simulink model "Driver"  (R2023b)
settings: Solver=FixedStepAuto  StartTime=0.0  StopTime=10.0  FixedStep=dt  RelTol=1e-3
undefined symbols (not defined in the file): lookAheadDistance, lowpassT, steerLockDeg, torqueLimit, trackReference
libraries: slpidlib x3, simulink_extras x2, eeGeneralControl x1
settings Model: Creator=lukec  LastModifiedBy=lukec

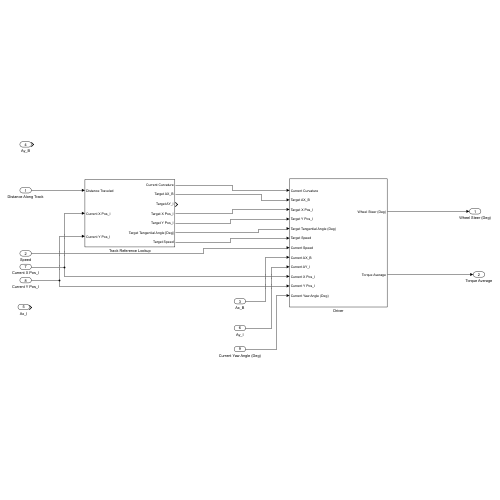
[thumbnail: Simulink's stored preview of the top-level diagram]
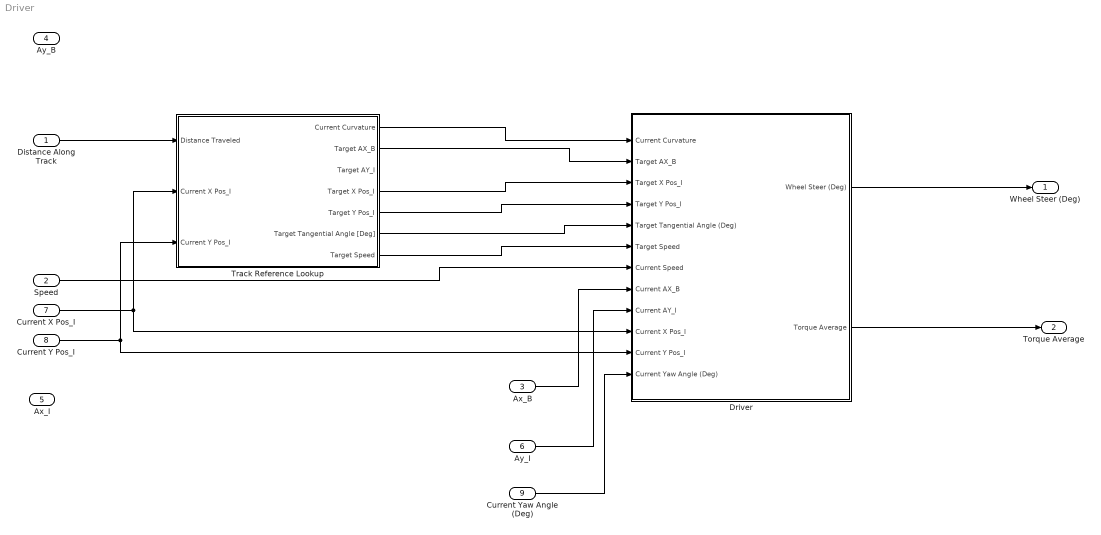
== system Driver ==
  Distance Along Track : Inport
  Speed : Inport  Port=2
  Ax_B : Inport  Port=3
  Ay_B : Inport  Port=4
  Ax_I : Inport  Port=5
  Ay_I : Inport  Port=6
  Current X Pos_I : Inport  Port=7
  Current Y Pos_I : Inport  Port=8
  Current Yaw Angle (Deg) : Inport  Port=9
  Driver : Subsystem
  Track Reference Lookup : Subsystem
  Wheel Steer (Deg) : Outport
  Torque Average : Outport  Port=2
  wires:
  Driver/1(Wheel Steer (Deg)) -> Wheel Steer (Deg)/1
  Track Reference Lookup/1(Current Curvature) -> Driver/1(Current Curvature)
  Track Reference Lookup/2(Target AX_B) -> Driver/2(Target AX_B)
  Track Reference Lookup/4(Target X Pos_I) -> Driver/3(Target X Pos_I)
  Track Reference Lookup/5(Target Y Pos_I) -> Driver/4(Target Y Pos_I)
  Distance Along Track/1 -> Track Reference Lookup/1(Distance Traveled)
  Ax_B/1 -> Driver/8(Current AX_B)
  Ay_I/1 -> Driver/9(Current AY_I)
  Current X Pos_I/1 -> Track Reference Lookup/2(Current X Pos_I), Driver/10(Current X Pos_I)
  Current Y Pos_I/1 -> Track Reference Lookup/3(Current Y Pos_I), Driver/11(Current Y Pos_I)
  Current Yaw Angle (Deg)/1 -> Driver/12(Current Yaw Angle (Deg))
  Track Reference Lookup/6(Target Tangential Angle [Deg]) -> Driver/5(Target Tangential Angle (Deg))
  Speed/1 -> Driver/7(Current Speed)
  Track Reference Lookup/7(Target Speed) -> Driver/6(Target Speed)
  Driver/2(Torque Average) -> Torque Average/1

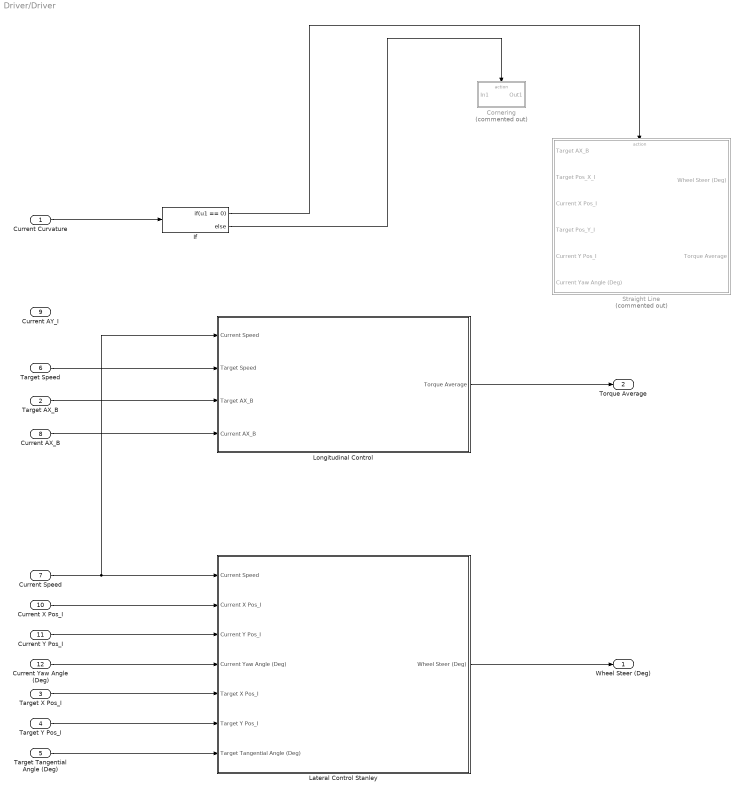
== system Driver/Driver ==
  Current Curvature : Inport
  Target AX_B : Inport  Port=2
  Target X Pos_I : Inport  Port=3
  Target Y Pos_I : Inport  Port=4
  Target Tangential Angle (Deg) : Inport  Port=5
  Target Speed : Inport  Port=6
  Current Speed : Inport  Port=7
  Current AX_B : Inport  Port=8
  Current AY_I : Inport  Port=9
  Current X Pos_I : Inport  Port=10
  Current Y Pos_I : Inport  Port=11
  Current Yaw Angle (Deg) : Inport  Port=12
  Cornering : Subsystem  Commented=on  TreatAsAtomicUnit=on
  If : If  IfExpression=u1 == 0
  Lateral Control Stanley : Subsystem
  Longitudinal Control : Subsystem
  Straight Line : Subsystem  Commented=on  TreatAsAtomicUnit=on
  Wheel Steer (Deg) : Outport
  Torque Average : Outport  Port=2
  wires:
  Current Curvature/1 -> If/1
  If/1 -> Straight Line/Action
  If/2 -> Cornering/Action
  Target X Pos_I/1 -> Lateral Control Stanley/5(Target X Pos_I)
  Target Y Pos_I/1 -> Lateral Control Stanley/6(Target Y Pos_I)
  Current X Pos_I/1 -> Lateral Control Stanley/2(Current X Pos_I)
  Current Y Pos_I/1 -> Lateral Control Stanley/3(Current Y Pos_I)
  Current Yaw Angle (Deg)/1 -> Lateral Control Stanley/4(Current Yaw Angle (Deg))
  Target Tangential Angle (Deg)/1 -> Lateral Control Stanley/7(Target Tangential Angle (Deg))
  Current Speed/1 -> Longitudinal Control/1(Current Speed), Lateral Control Stanley/1(Current Speed)
  Lateral Control Stanley/1(Wheel Steer (Deg)) -> Wheel Steer (Deg)/1
  Longitudinal Control/1(Torque Average) -> Torque Average/1
  Target Speed/1 -> Longitudinal Control/2(Target Speed)
  Current AX_B/1 -> Longitudinal Control/4(Current AX_B)
  Target AX_B/1 -> Longitudinal Control/3(Target AX_B)

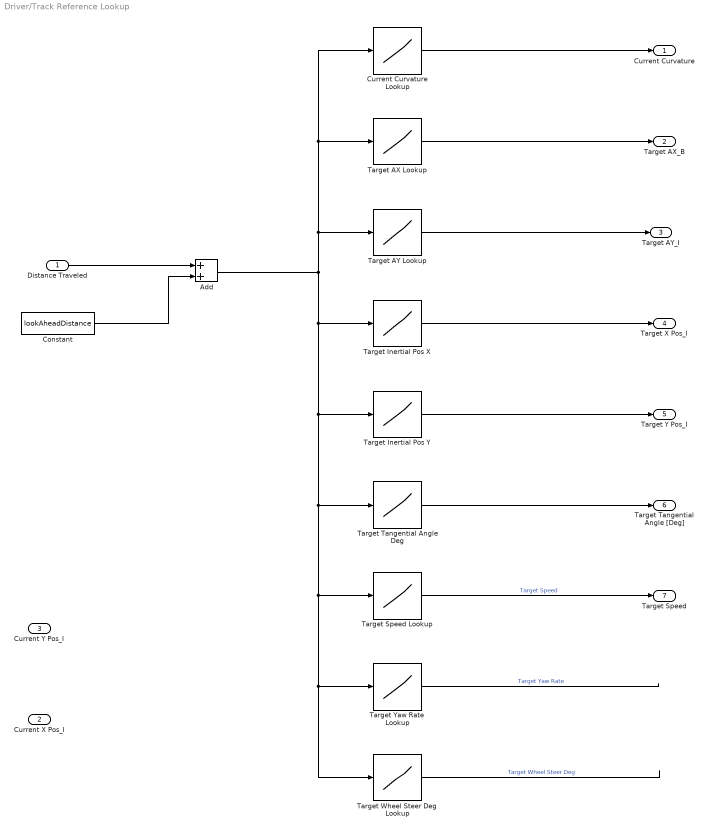
== system Driver/Track Reference Lookup ==
  Distance Traveled : Inport
  Current X Pos_I : Inport  Port=2
  Current Y Pos_I : Inport  Port=3
  Add : Sum
  Constant : Constant  Value=lookAheadDistance
  Current Curvature Lookup : Lookup_n-D  NumberOfTableDimensions=1  BreakpointsForDimension1=trackReference.posAlongTrack  Table=trackReference.curvature  InternalRulePriority=Speed  RndMeth=Simplest
  Target AX Lookup : Lookup_n-D  NumberOfTableDimensions=1  BreakpointsForDimension1=trackReference.posAlongTrack  Table=trackReference.AX  InternalRulePriority=Speed  RndMeth=Simplest
  Target AY Lookup : Lookup_n-D  NumberOfTableDimensions=1  BreakpointsForDimension1=trackReference.posAlongTrack  Table=trackReference.AY  InternalRulePriority=Speed  RndMeth=Simplest
  Target Inertial Pos X : Lookup_n-D  NumberOfTableDimensions=1  BreakpointsForDimension1=trackReference.posAlongTrack  Table=trackReference.X  InternalRulePriority=Speed  RndMeth=Simplest
  Target Inertial Pos Y : Lookup_n-D  NumberOfTableDimensions=1  BreakpointsForDimension1=trackReference.posAlongTrack  Table=trackReference.Y  InternalRulePriority=Speed  RndMeth=Simplest
  Target Speed Lookup : Lookup_n-D  NumberOfTableDimensions=1  BreakpointsForDimension1=trackReference.posAlongTrack  Table=[trackReference.speed(2); trackReference.speed(2:end)]  InternalRulePriority=Speed  RndMeth=Simplest
  Target Tangential Angle Deg : Lookup_n-D  NumberOfTableDimensions=1  BreakpointsForDimension1=trackReference.posAlongTrack  Table=trackReference.tangentialAngDeg  InternalRulePriority=Speed  RndMeth=Simplest
  Target Wheel Steer Deg Lookup : Lookup_n-D  NumberOfTableDimensions=1  BreakpointsForDimension1=trackReference.posAlongTrack  Table=trackReference.wheelSteerDeg  InternalRulePriority=Speed  RndMeth=Simplest
  Target Yaw Rate Lookup : Lookup_n-D  NumberOfTableDimensions=1  BreakpointsForDimension1=trackReference.posAlongTrack  Table=trackReference.yawRate  InternalRulePriority=Speed  RndMeth=Simplest
  Current Curvature : Outport
  Target AX_B : Outport  Port=2
  Target AY_I : Outport  Port=3
  Target X Pos_I : Outport  Port=4
  Target Y Pos_I : Outport  Port=5
  Target Tangential Angle [Deg] : Outport  Port=6
  Target Speed : Outport  Port=7
  wires:
  Distance Traveled/1 -> Add/1
  Target AY Lookup/1 -> Target AY_I/1
  Current Curvature Lookup/1 -> Current Curvature/1
  Target AX Lookup/1 -> Target AX_B/1
  Target Inertial Pos X/1 -> Target X Pos_I/1
  Target Inertial Pos Y/1 -> Target Y Pos_I/1
  Target Tangential Angle Deg/1 -> Target Tangential Angle [Deg]/1
  Target Speed Lookup/1 -> Target Speed/1  "Target Speed"
  Add/1 -> Target AY Lookup/1, Target AX Lookup/1, Current Curvature Lookup/1, Target Wheel Steer Deg Lookup/1, Target Yaw Rate Lookup/1, Target Speed Lookup/1, Target Tangential Angle Deg/1, Target Inertial Pos Y/1, Target Inertial Pos X/1
  Constant/1 -> Add/2
  Target Yaw Rate Lookup/1 -> ?  "Target Yaw Rate"
  Target Wheel Steer Deg Lookup/1 -> ?  "Target Wheel Steer Deg"

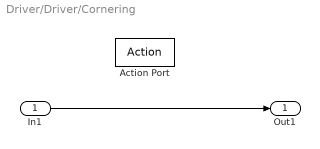
== system Driver/Driver/Cornering ==
  In1 : Inport
  Action Port : ActionPort  ActionPortLabel=else
  Out1 : Outport
  wires:
  In1/1 -> Out1/1

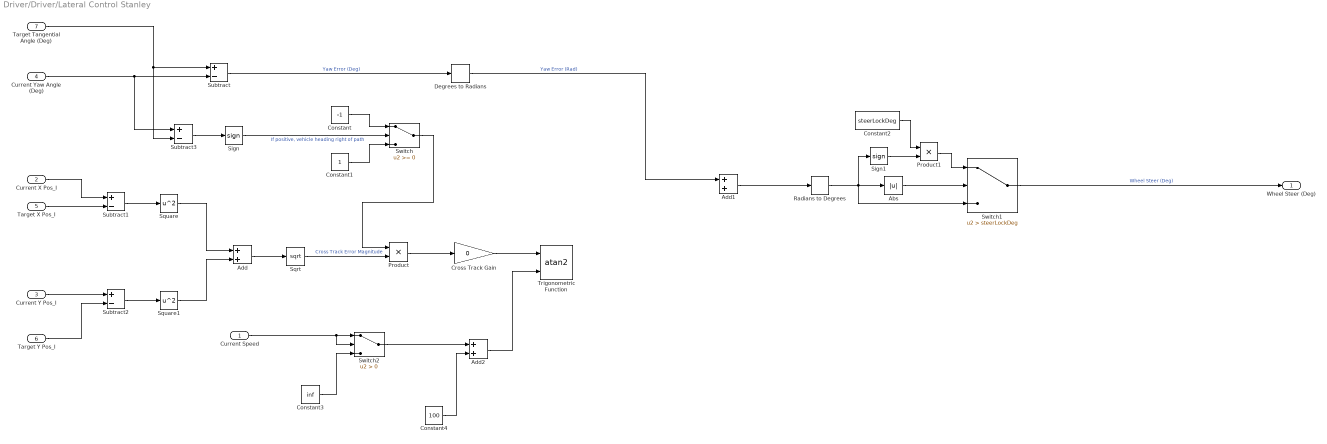
== system Driver/Driver/Lateral Control Stanley ==
  Current Speed : Inport
  Current X Pos_I : Inport  Port=2
  Current Y Pos_I : Inport  Port=3
  Current Yaw Angle (Deg) : Inport  Port=4
  Target X Pos_I : Inport  Port=5
  Target Y Pos_I : Inport  Port=6
  Target Tangential Angle (Deg) : Inport  Port=7
  Abs : Abs  SaturateOnIntegerOverflow=off
  Add : Sum
  Add1 : Sum
  Add2 : Sum
  Constant : Constant  Value=-1
  Constant1 : Constant
  Constant2 : Constant  Value=steerLockDeg
  Constant3 : Constant  Value=inf
  Constant4 : Constant  Value=100
  Cross Track Gain : Gain  Gain=0
  Degrees to Radians : simulink_extras/Transformations/Degrees to Radians
  Product : Product
  Product1 : Product
  Radians to Degrees : simulink_extras/Transformations/Radians to Degrees
  Sign : Signum
  Sign1 : Signum
  Sqrt : Sqrt
  Square : Math  Operator=square
  Square1 : Math  Operator=square
  Subtract{,1..3} (4 alike) : Sum  Inputs=+-
  Switch : Switch  SaturateOnIntegerOverflow=off  InputSameDT=off
  Switch1 : Switch  Criteria=u2 > Threshold  Threshold=steerLockDeg  SaturateOnIntegerOverflow=off  InputSameDT=off
  Switch2 : Switch  Criteria=u2 > Threshold  SaturateOnIntegerOverflow=off  InputSameDT=off
  Trigonometric Function : Trigonometry  Operator=atan2
  Wheel Steer (Deg) : Outport
  wires:
  Target Tangential Angle (Deg)/1 -> Subtract3/2, Subtract/1
  Current Yaw Angle (Deg)/1 -> Subtract3/1, Subtract/2
  Subtract/1 -> Degrees to Radians/1  "Yaw Error (Deg)"
  Current X Pos_I/1 -> Subtract1/1
  Target X Pos_I/1 -> Subtract1/2
  Subtract1/1 -> Square/1
  Current Y Pos_I/1 -> Subtract2/1
  Target Y Pos_I/1 -> Subtract2/2
  Subtract2/1 -> Square1/1
  Square/1 -> Add/1
  Square1/1 -> Add/2
  Add/1 -> Sqrt/1
  Cross Track Gain/1 -> Trigonometric Function/1
  Subtract3/1 -> Sign/1
  Sign/1 -> Switch/2  "If positive, vehicle heading right of path"
  Constant/1 -> Switch/1
  Constant1/1 -> Switch/3
  Sqrt/1 -> Product/2  "Cross Track Error Magnitude"
  Switch/1 -> Product/1
  Product/1 -> Cross Track Gain/1
  Degrees to Radians/1 -> Add1/1  "Yaw Error (Rad)"
  Add1/1 -> Radians to Degrees/1
  Radians to Degrees/1 -> Sign1/1, Switch1/3, Abs/1
  Current Speed/1 -> Switch2/2, Switch2/1
  Abs/1 -> Switch1/2
  Constant2/1 -> Product1/1
  Sign1/1 -> Product1/2
  Product1/1 -> Switch1/1
  Switch1/1 -> Wheel Steer (Deg)/1  "Wheel Steer (Deg)"
  Constant3/1 -> Switch2/3
  Switch2/1 -> Add2/1
  Add2/1 -> Trigonometric Function/2
  Constant4/1 -> Add2/2

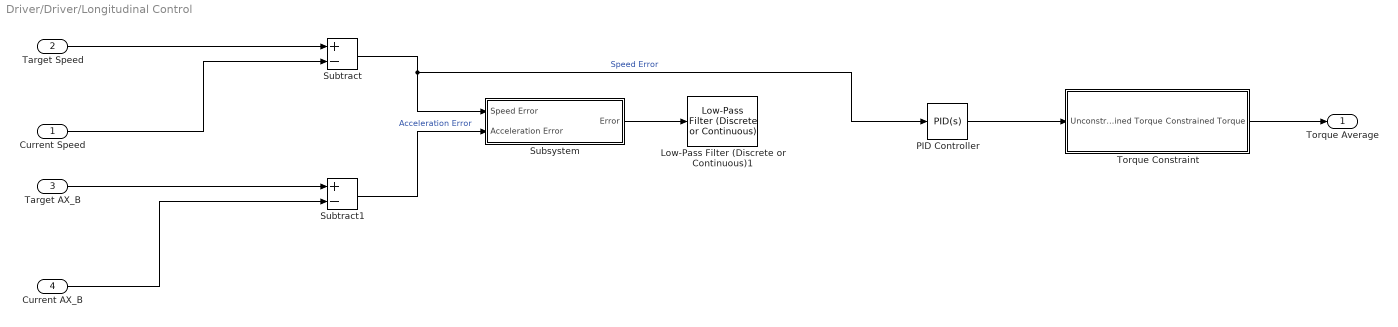
== system Driver/Driver/Longitudinal Control ==
  Current Speed : Inport
  Target Speed : Inport  Port=2
  Target AX_B : Inport  Port=3
  Current AX_B : Inport  Port=4
  Low-Pass Filter (Discrete or Continuous)1 : eeGeneralControl/Low-Pass Filter (Discrete or Continuous)  K=1  T=lowpassT  B=inf  A=-inf  init_option=Inherited from block input  x0=0  Ts=-1
  PID Controller : slpidlib/PID Controller  Controller=PID  Form=Parallel  TimeDomain=Continuous-time  UseExternalTs=off  SampleTime=-1  IntegratorMethod=Forward Euler  FilterMethod=Forward Euler  ControllerParametersSource=internal  P=5  I=1  UseKiTs=off  D=1  N=100  UseFilter=on  TunerSelectOption=Transfer Function Based (PID Tuner App)  InitialConditionSource=internal  InitialConditionForIntegrator=0  InitialConditionForFilter=0  DifferentiatorICPrevScaledInput=0  ExternalReset=none  TrackingMode=off  Kt=1  LimitOutput=off  SatLimitsSource=internal  UpperSaturationLimit=inf  LowerSaturationLimit=-inf  LinearizeAsGain=on  AntiWindupMode=none  Kb=1  LimitIntegrator=off  UpperIntegratorSaturationLimit=inf  LowerIntegratorSaturationLimit=-inf  POutMin=[]  POutMax=[]  IOutMin=[]  IOutMax=[]  DOutMin=[]  DOutMax=[]  NOutMin=[]  NOutMax=[]  SumOutMin=[]  SumOutMax=[]  SaturationOutMin=[]  SaturationOutMax=[]  PParamMin=[]  PParamMax=[]  IParamMin=[]  IParamMax=[]  DParamMin=[]  DParamMax=[]  NParamMin=[]  NParamMax=[]  KbParamMin=[]  KbParamMax=[]  KtParamMin=[]  KtParamMax=[]  KbOutMin=[]  KbOutMax=[]  KtOutMin=[]  KtOutMax=[]  IntegratorOutMin=[]  IntegratorOutMax=[]  FilterOutMin=[]  FilterOutMax=[]  SumI1OutMin=[]  SumI1OutMax=[]  SumI2OutMin=[]  SumI2OutMax=[]  SumI3OutMin=[]  SumI3OutMax=[]  SumI4OutMin=[]  SumI4OutMax=[]  SumDOutMin=[]  SumDOutMax=[]  DifferentiatorOutMin=[]  DifferentiatorOutMax=[]  FilterDiffOutCoefMin=[]  FilterDiffOutCoefMax=[]  ReciprocalOutMin=[]  ReciprocalOutMax=[]  SumDenOutMin=[]  SumDenOutMax=[]  SumNumOutMin=[]  SumNumOutMax=[]  DivideOutMin=[]  DivideOutMax=[]  UdiffTsProdOutMin=[]  UdiffTsProdOutMax=[]  NTsProdOutMin=[]  NTsProdOutMax=[]  UintegralTsProdOutMin=[]  UintegralTsProdOutMax=[]  UngainTsProdOutMin=[]  UngainTsProdOutMax=[]  ClampingZeroOutDataTypeStr=Inherit: Inherit via back propagation  ClampingZeroOutMin=[]  ClampingZeroOutMax=[]  FilterDenConstantOutDataTypeStr=Inherit: Inherit via back propagation  FilterDenConstantOutMin=[]  FilterDenConstantOutMax=[]  PCopyOutDataTypeStr=Inherit: Inherit via back propagation  PCopyOutMin=[]  PCopyOutMax=[]  NCopyOutDataTypeStr=Inherit: Inherit via back propagation  NCopyOutMin=[]  NCopyOutMax=[]  IntegratorContinuousStateAttributes=''  IntegratorStateMustResolveToSignalObject=off  IntegratorRTWStateStorageClass=Auto  FilterContinuousStateAttributes=''  FilterStateMustResolveToSignalObject=off  FilterRTWStateStorageClass=Auto  ParallelPVariant=InternalParameters  IdealPVariant=Disabled  IVariant=InternalParameters  DVariant=InternalParameters  IntegratorVariant=Continuous  SatVariant=Disabled  AWVariant=Passthrough  PCopyVariant=Disabled  TRVariant=Disabled  FdbkBlocksVariant=Forward  IdealPFdbkVariant=Disabled  SatFdbkVariant=Disabled  DerivativeFilterVariant=ContFilter  NVariant=InternalParameters  NCopyVariant=Disabled  FilterICVariant=InternalICsFilter  IntegratorICVariant=InternalICs  ExternalResetVariant=Disabled  TRSumVariant=Passthrough  SumFdbkVariant=Disabled  SumVariant=Sum_PID  TsampFilterVariant=InternalTs  TsampNgainVariant=Passthrough  TsampIntegralVariant=Disabled_SignalSpec  ExternalSaturationOutDataTypeStr=Inherit: Same as second input
  Subsystem : Subsystem
  Subtract : Sum  Inputs=+-
  Subtract1 : Sum  Inputs=+-
  Torque Constraint : Subsystem
  Torque Average : Outport
  wires:
  Target Speed/1 -> Subtract/1
  Current Speed/1 -> Subtract/2
  PID Controller/1 -> Torque Constraint/1(Unconstrained Torque)
  Target AX_B/1 -> Subtract1/1
  Current AX_B/1 -> Subtract1/2
  Torque Constraint/1(Constrained Torque) -> Torque Average/1
  Subsystem/1(Error) -> Low-Pass Filter (Discrete or Continuous)1/1
  Subtract/1 -> PID Controller/1, Subsystem/1(Speed Error)  "Speed Error"
  Subtract1/1 -> Subsystem/2(Acceleration Error)  "Acceleration Error"

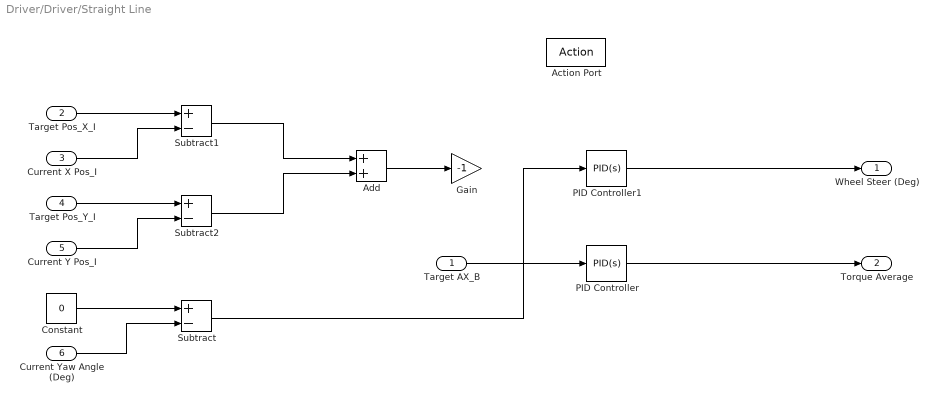
== system Driver/Driver/Straight Line ==
  Target AX_B : Inport
  Target Pos_X_I : Inport  Port=2
  Current X Pos_I : Inport  Port=3
  Target Pos_Y_I : Inport  Port=4
  Current Y Pos_I : Inport  Port=5
  Current Yaw Angle (Deg) : Inport  Port=6
  Action Port : ActionPort  ActionPortLabel=if(u1 == 0)
  Add : Sum
  Constant : Constant  Value=0
  Gain : Gain  Gain=-1
  PID Controller : slpidlib/PID Controller  Controller=PID  Form=Parallel  TimeDomain=Continuous-time  UseExternalTs=off  SampleTime=-1  IntegratorMethod=Forward Euler  FilterMethod=Forward Euler  ControllerParametersSource=internal  P=1  I=1  UseKiTs=off  D=0  N=100  UseFilter=on  TunerSelectOption=Transfer Function Based (PID Tuner App)  InitialConditionSource=internal  InitialConditionForIntegrator=0  InitialConditionForFilter=0  DifferentiatorICPrevScaledInput=0  ExternalReset=none  TrackingMode=off  Kt=1  LimitOutput=off  SatLimitsSource=internal  UpperSaturationLimit=inf  LowerSaturationLimit=-inf  LinearizeAsGain=on  AntiWindupMode=none  Kb=1  LimitIntegrator=off  UpperIntegratorSaturationLimit=inf  LowerIntegratorSaturationLimit=-inf  POutMin=[]  POutMax=[]  IOutMin=[]  IOutMax=[]  DOutMin=[]  DOutMax=[]  NOutMin=[]  NOutMax=[]  SumOutMin=[]  SumOutMax=[]  SaturationOutMin=[]  SaturationOutMax=[]  PParamMin=[]  PParamMax=[]  IParamMin=[]  IParamMax=[]  DParamMin=[]  DParamMax=[]  NParamMin=[]  NParamMax=[]  KbParamMin=[]  KbParamMax=[]  KtParamMin=[]  KtParamMax=[]  KbOutMin=[]  KbOutMax=[]  KtOutMin=[]  KtOutMax=[]  IntegratorOutMin=[]  IntegratorOutMax=[]  FilterOutMin=[]  FilterOutMax=[]  SumI1OutMin=[]  SumI1OutMax=[]  SumI2OutMin=[]  SumI2OutMax=[]  SumI3OutMin=[]  SumI3OutMax=[]  SumI4OutMin=[]  SumI4OutMax=[]  SumDOutMin=[]  SumDOutMax=[]  DifferentiatorOutMin=[]  DifferentiatorOutMax=[]  FilterDiffOutCoefMin=[]  FilterDiffOutCoefMax=[]  ReciprocalOutMin=[]  ReciprocalOutMax=[]  SumDenOutMin=[]  SumDenOutMax=[]  SumNumOutMin=[]  SumNumOutMax=[]  DivideOutMin=[]  DivideOutMax=[]  UdiffTsProdOutMin=[]  UdiffTsProdOutMax=[]  NTsProdOutMin=[]  NTsProdOutMax=[]  UintegralTsProdOutMin=[]  UintegralTsProdOutMax=[]  UngainTsProdOutMin=[]  UngainTsProdOutMax=[]  ClampingZeroOutDataTypeStr=Inherit: Inherit via back propagation  ClampingZeroOutMin=[]  ClampingZeroOutMax=[]  FilterDenConstantOutDataTypeStr=Inherit: Inherit via back propagation  FilterDenConstantOutMin=[]  FilterDenConstantOutMax=[]  PCopyOutDataTypeStr=Inherit: Inherit via back propagation  PCopyOutMin=[]  PCopyOutMax=[]  NCopyOutDataTypeStr=Inherit: Inherit via back propagation  NCopyOutMin=[]  NCopyOutMax=[]  IntegratorContinuousStateAttributes=''  IntegratorStateMustResolveToSignalObject=off  IntegratorRTWStateStorageClass=Auto  FilterContinuousStateAttributes=''  FilterStateMustResolveToSignalObject=off  FilterRTWStateStorageClass=Auto  ParallelPVariant=InternalParameters  IdealPVariant=Disabled  IVariant=InternalParameters  DVariant=InternalParameters  IntegratorVariant=Continuous  SatVariant=Disabled  AWVariant=Passthrough  PCopyVariant=Disabled  TRVariant=Disabled  FdbkBlocksVariant=Forward  IdealPFdbkVariant=Disabled  SatFdbkVariant=Disabled  DerivativeFilterVariant=ContFilter  NVariant=InternalParameters  NCopyVariant=Disabled  FilterICVariant=InternalICsFilter  IntegratorICVariant=InternalICs  ExternalResetVariant=Disabled  TRSumVariant=Passthrough  SumFdbkVariant=Disabled  SumVariant=Sum_PID  TsampFilterVariant=InternalTs  TsampNgainVariant=Passthrough  TsampIntegralVariant=Disabled_SignalSpec  ExternalSaturationOutDataTypeStr=Inherit: Same as second input
  PID Controller1 : slpidlib/PID Controller  Controller=PID  Form=Parallel  TimeDomain=Continuous-time  UseExternalTs=off  SampleTime=-1  IntegratorMethod=Forward Euler  FilterMethod=Forward Euler  ControllerParametersSource=internal  P=2  I=5  UseKiTs=off  D=0  N=100  UseFilter=on  TunerSelectOption=Transfer Function Based (PID Tuner App)  InitialConditionSource=internal  InitialConditionForIntegrator=0  InitialConditionForFilter=0  DifferentiatorICPrevScaledInput=0  ExternalReset=none  TrackingMode=off  Kt=1  LimitOutput=off  SatLimitsSource=internal  UpperSaturationLimit=inf  LowerSaturationLimit=-inf  LinearizeAsGain=on  AntiWindupMode=none  Kb=1  LimitIntegrator=off  UpperIntegratorSaturationLimit=inf  LowerIntegratorSaturationLimit=-inf  POutMin=[]  POutMax=[]  IOutMin=[]  IOutMax=[]  DOutMin=[]  DOutMax=[]  NOutMin=[]  NOutMax=[]  SumOutMin=[]  SumOutMax=[]  SaturationOutMin=[]  SaturationOutMax=[]  PParamMin=[]  PParamMax=[]  IParamMin=[]  IParamMax=[]  DParamMin=[]  DParamMax=[]  NParamMin=[]  NParamMax=[]  KbParamMin=[]  KbParamMax=[]  KtParamMin=[]  KtParamMax=[]  KbOutMin=[]  KbOutMax=[]  KtOutMin=[]  KtOutMax=[]  IntegratorOutMin=[]  IntegratorOutMax=[]  FilterOutMin=[]  FilterOutMax=[]  SumI1OutMin=[]  SumI1OutMax=[]  SumI2OutMin=[]  SumI2OutMax=[]  SumI3OutMin=[]  SumI3OutMax=[]  SumI4OutMin=[]  SumI4OutMax=[]  SumDOutMin=[]  SumDOutMax=[]  DifferentiatorOutMin=[]  DifferentiatorOutMax=[]  FilterDiffOutCoefMin=[]  FilterDiffOutCoefMax=[]  ReciprocalOutMin=[]  ReciprocalOutMax=[]  SumDenOutMin=[]  SumDenOutMax=[]  SumNumOutMin=[]  SumNumOutMax=[]  DivideOutMin=[]  DivideOutMax=[]  UdiffTsProdOutMin=[]  UdiffTsProdOutMax=[]  NTsProdOutMin=[]  NTsProdOutMax=[]  UintegralTsProdOutMin=[]  UintegralTsProdOutMax=[]  UngainTsProdOutMin=[]  UngainTsProdOutMax=[]  ClampingZeroOutDataTypeStr=Inherit: Inherit via back propagation  ClampingZeroOutMin=[]  ClampingZeroOutMax=[]  FilterDenConstantOutDataTypeStr=Inherit: Inherit via back propagation  FilterDenConstantOutMin=[]  FilterDenConstantOutMax=[]  PCopyOutDataTypeStr=Inherit: Inherit via back propagation  PCopyOutMin=[]  PCopyOutMax=[]  NCopyOutDataTypeStr=Inherit: Inherit via back propagation  NCopyOutMin=[]  NCopyOutMax=[]  IntegratorContinuousStateAttributes=''  IntegratorStateMustResolveToSignalObject=off  IntegratorRTWStateStorageClass=Auto  FilterContinuousStateAttributes=''  FilterStateMustResolveToSignalObject=off  FilterRTWStateStorageClass=Auto  ParallelPVariant=InternalParameters  IdealPVariant=Disabled  IVariant=InternalParameters  DVariant=InternalParameters  IntegratorVariant=Continuous  SatVariant=Disabled  AWVariant=Passthrough  PCopyVariant=Disabled  TRVariant=Disabled  FdbkBlocksVariant=Forward  IdealPFdbkVariant=Disabled  SatFdbkVariant=Disabled  DerivativeFilterVariant=ContFilter  NVariant=InternalParameters  NCopyVariant=Disabled  FilterICVariant=InternalICsFilter  IntegratorICVariant=InternalICs  ExternalResetVariant=Disabled  TRSumVariant=Passthrough  SumFdbkVariant=Disabled  SumVariant=Sum_PID  TsampFilterVariant=InternalTs  TsampNgainVariant=Passthrough  TsampIntegralVariant=Disabled_SignalSpec  ExternalSaturationOutDataTypeStr=Inherit: Same as second input
  Subtract : Sum  Inputs=+-
  Subtract1 : Sum  Inputs=+-
  Subtract2 : Sum  Inputs=+-
  Wheel Steer (Deg) : Outport
  Torque Average : Outport  Port=2
  wires:
  Target AX_B/1 -> PID Controller/1
  PID Controller/1 -> Torque Average/1
  Target Pos_X_I/1 -> Subtract1/1
  Current X Pos_I/1 -> Subtract1/2
  Target Pos_Y_I/1 -> Subtract2/1
  Current Y Pos_I/1 -> Subtract2/2
  Subtract1/1 -> Add/1
  Subtract2/1 -> Add/2
  PID Controller1/1 -> Wheel Steer (Deg)/1
  Add/1 -> Gain/1
  Constant/1 -> Subtract/1
  Current Yaw Angle (Deg)/1 -> Subtract/2
  Subtract/1 -> PID Controller1/1

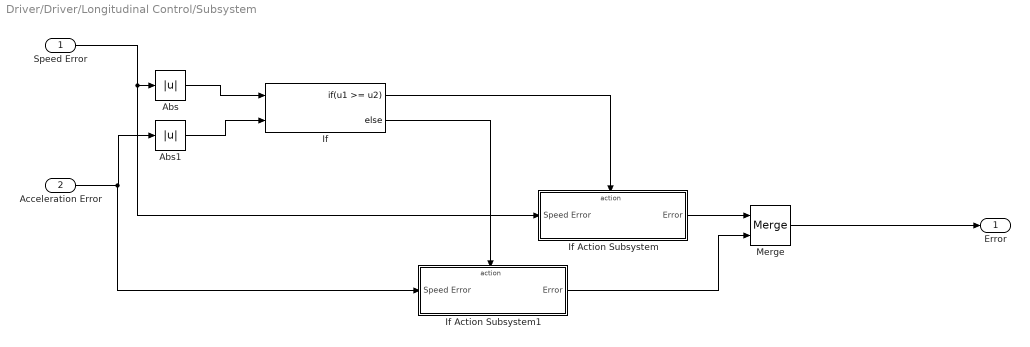
== system Driver/Driver/Longitudinal Control/Subsystem ==
  Speed Error : Inport
  Acceleration Error : Inport  Port=2
  Abs : Abs  SaturateOnIntegerOverflow=off
  Abs1 : Abs  SaturateOnIntegerOverflow=off
  If : If  NumInputs=2  IfExpression=u1 >= u2
  If Action Subsystem : Subsystem  TreatAsAtomicUnit=on
  If Action Subsystem1 : Subsystem  TreatAsAtomicUnit=on
  Merge : Merge
  Error : Outport
  wires:
  Speed Error/1 -> If Action Subsystem/1(Speed Error), Abs/1
  If Action Subsystem1/1(Error) -> Merge/2
  Acceleration Error/1 -> If Action Subsystem1/1(Speed Error), Abs1/1
  Abs/1 -> If/1
  If/1 -> If Action Subsystem/Action
  If Action Subsystem/1(Error) -> Merge/1
  Abs1/1 -> If/2
  If/2 -> If Action Subsystem1/Action
  Merge/1 -> Error/1

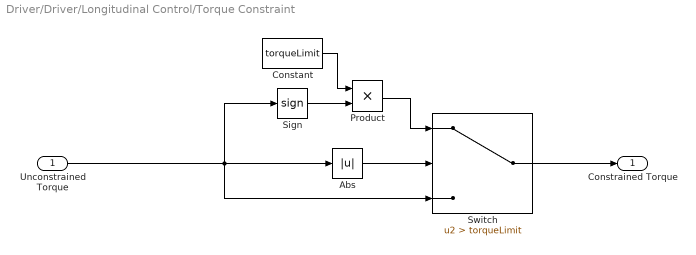
== system Driver/Driver/Longitudinal Control/Torque Constraint ==
  Unconstrained Torque : Inport
  Abs : Abs  SaturateOnIntegerOverflow=off
  Constant : Constant  Value=torqueLimit
  Product : Product
  Sign : Signum
  Switch : Switch  Criteria=u2 > Threshold  Threshold=torqueLimit  SaturateOnIntegerOverflow=off  InputSameDT=off
  Constrained Torque : Outport
  wires:
  Sign/1 -> Product/2
  Constant/1 -> Product/1
  Product/1 -> Switch/1
  Unconstrained Torque/1 -> Switch/3, Sign/1, Abs/1
  Switch/1 -> Constrained Torque/1
  Abs/1 -> Switch/2

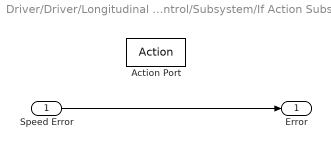
== system Driver/Driver/Longitudinal Control/Subsystem/If Action Subsystem ==
  Speed Error : Inport
  Action Port : ActionPort  ActionPortLabel=if(u1 >= u2)
  Error : Outport
  wires:
  Speed Error/1 -> Error/1

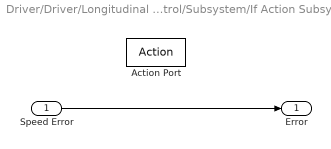
== system Driver/Driver/Longitudinal Control/Subsystem/If Action Subsystem1 ==
  Speed Error : Inport
  Action Port : ActionPort  ActionPortLabel=else
  Error : Outport
  wires:
  Speed Error/1 -> Error/1
